simulink model "DistanceCal"  (R2022b)
settings: Solver=VariableStepAuto  StartTime=0.0  StopTime=1.0  RelTol=1e-3
settings Model: Creator=ADMIN  LastModifiedBy=ADMIN

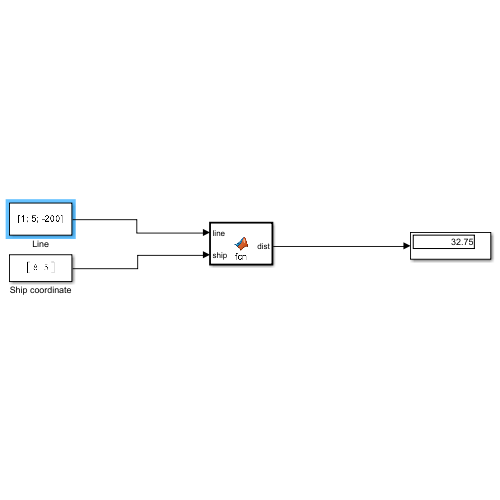
[thumbnail: Simulink's stored preview of the top-level diagram]
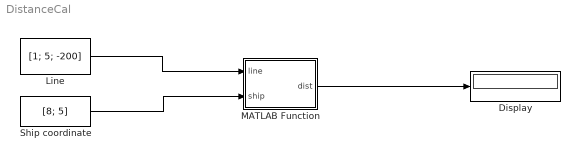
== system DistanceCal ==
  Display : Display
  Line : Constant  Value=[1; 5; -200]
  MATLAB Function : MATLAB Function  TreatAsAtomicUnit=on
  Ship coordinate : Constant  Value=[8; 5]
  wires:
  Line/1 -> MATLAB Function/1(line)
  Ship coordinate/1 -> MATLAB Function/2(ship)
  MATLAB Function/1(dist) -> Display/1

== matlab function DistanceCal/MATLAB Function ==
  data: line input; dist output; ship input
function dist = fcn(line,ship)

dist = abs(line(1)*ship(1) + line(2)*ship(2) + line(3)) / hypot(line(1),line(2));
